simulink model "StateMachine_v3"  (R2015a)
settings: Solver=ode1  StartTime=0.0  StopTime=Inf  FixedStep=0.001  RelTol=1e-3
PostLoadFcn:
  | , if any(exist('dsrtsu_mdlpostloadfcn', 'file') == [2, 3, 6]), try dsrtsu_mdlpostloadfcn('Execute', bdroot); catch fprintf('Error in PostLoadFcn (dsrtsu_mdlpostloadfcn) for model "%s":\n %s\n', bdroot, lasterr); end, end,
libraries: rtican x25, rti1401lib_adc_type4 x16, rti1401lib_dio_type3 x16, rtilib1401 x1
(part 6 of 6)

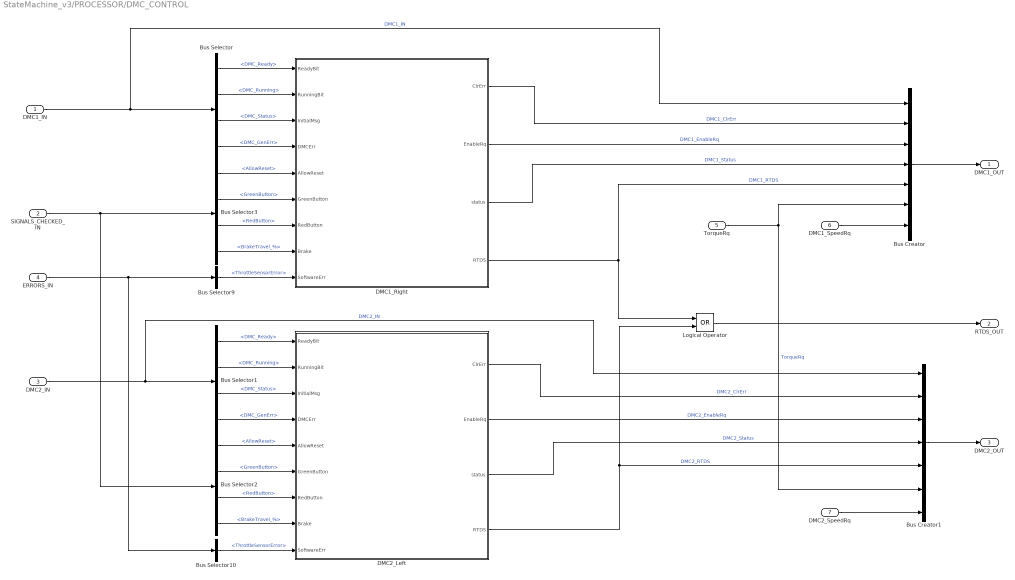
== system StateMachine_v3/PROCESSOR/DMC_CONTROL ==
  DMC1_IN : Inport
  SIGNALS_CHECKED_IN : Inport  Port=2
  DMC2_IN : Inport  Port=3
  ERRORS_IN : Inport  Port=4
  TorqueRq : Inport  Port=5
  DMC1_SpeedRq : Inport  Port=6
  DMC2_SpeedRq : Inport  Port=7
  Bus Creator : BusCreator  Inputs=7
  Bus Creator1 : BusCreator  Inputs=7
  Bus Selector : BusSelector  OutputSignals=DMC_Ready,DMC_Running,DMC_Status,DMC_GenErr
  Bus Selector1 : BusSelector  OutputSignals=DMC_Ready,DMC_Running,DMC_Status,DMC_GenErr
  Bus Selector10 : BusSelector  OutputSignals=ThrottleSensorError
  Bus Selector2 : BusSelector  OutputSignals=SIGNALS.OtherInputs.AllowReset,SIGNALS.DigitalInputs.GreenButton,SIGNALS.DigitalInputs.RedButton,BrakeTravel_%
  Bus Selector3 : BusSelector  OutputSignals=SIGNALS.OtherInputs.AllowReset,SIGNALS.DigitalInputs.GreenButton,SIGNALS.DigitalInputs.RedButton,BrakeTravel_%
  Bus Selector9 : BusSelector  OutputSignals=ThrottleSensorError
  DMC1_Right : Stateflow chart  TreatAsAtomicUnit=on
  DMC2_Left : Stateflow chart  TreatAsAtomicUnit=on
  Logical Operator : Logic  Operator=OR  AllPortsSameDT=off  OutDataTypeStr=boolean
  DMC1_OUT : Outport
  RTDS_OUT : Outport  Port=2
  DMC2_OUT : Outport  Port=3
  wires:
  TorqueRq/1 -> Bus Creator1/6, Bus Creator/6  "TorqueRq"
  ERRORS_IN/1 -> Bus Selector10/1, Bus Selector9/1
  SIGNALS_CHECKED_IN/1 -> Bus Selector2/1, Bus Selector3/1
  DMC1_Right/3(status) -> Bus Creator/4  "DMC1_Status"
  Bus Creator/1 -> DMC1_OUT/1
  Bus Selector9/1 -> DMC1_Right/9(SoftwareErr)  "<ThrottleSensorError>"
  Bus Selector10/1 -> DMC2_Left/9(SoftwareErr)  "<ThrottleSensorError>"
  Bus Creator1/1 -> DMC2_OUT/1
  Bus Selector/4 -> DMC1_Right/4(DMCErr)  "<DMC_GenErr>"
  Bus Selector3/3 -> DMC1_Right/7(RedButton)  "<RedButton>"
  DMC2_IN/1 -> Bus Creator1/1, Bus Selector1/1  "DMC2_IN"
  Bus Selector1/4 -> DMC2_Left/4(DMCErr)  "<DMC_GenErr>"
  DMC1_SpeedRq/1 -> Bus Creator/7
  DMC2_Left/3(status) -> Bus Creator1/4  "DMC2_Status"
  Bus Selector2/4 -> DMC2_Left/8(Brake)  "<BrakeTravel_%>"
  DMC2_Left/4(RTDS) -> Bus Creator1/5, Logical Operator/2  "DMC2_RTDS"
  DMC1_Right/4(RTDS) -> Logical Operator/1, Bus Creator/5  "DMC1_RTDS"
  Logical Operator/1 -> RTDS_OUT/1
  DMC2_Left/1(ClrErr) -> Bus Creator1/2  "DMC2_ClrErr"
  Bus Selector2/1 -> DMC2_Left/5(AllowReset)  "<AllowReset>"
  Bus Selector1/2 -> DMC2_Left/2(RunningBit)  "<DMC_Running>"
  DMC1_IN/1 -> Bus Creator/1, Bus Selector/1  "DMC1_IN"
  DMC1_Right/1(ClrErr) -> Bus Creator/2  "DMC1_ClrErr"
  DMC2_SpeedRq/1 -> Bus Creator1/7
  Bus Selector1/1 -> DMC2_Left/1(ReadyBit)  "<DMC_Ready>"
  Bus Selector3/2 -> DMC1_Right/6(GreenButton)  "<GreenButton>"
  Bus Selector/3 -> DMC1_Right/3(InitialMsg)  "<DMC_Status>"
  Bus Selector1/3 -> DMC2_Left/3(InitialMsg)  "<DMC_Status>"
  Bus Selector/1 -> DMC1_Right/1(ReadyBit)  "<DMC_Ready>"
  Bus Selector3/4 -> DMC1_Right/8(Brake)  "<BrakeTravel_%>"
  Bus Selector2/3 -> DMC2_Left/7(RedButton)  "<RedButton>"
  DMC2_Left/2(EnableRq) -> Bus Creator1/3  "DMC2_EnableRq"
  Bus Selector/2 -> DMC1_Right/2(RunningBit)  "<DMC_Running>"
  Bus Selector2/2 -> DMC2_Left/6(GreenButton)  "<GreenButton>"
  Bus Selector3/1 -> DMC1_Right/5(AllowReset)  "<AllowReset>"
  DMC1_Right/2(EnableRq) -> Bus Creator/3  "DMC1_EnableRq"

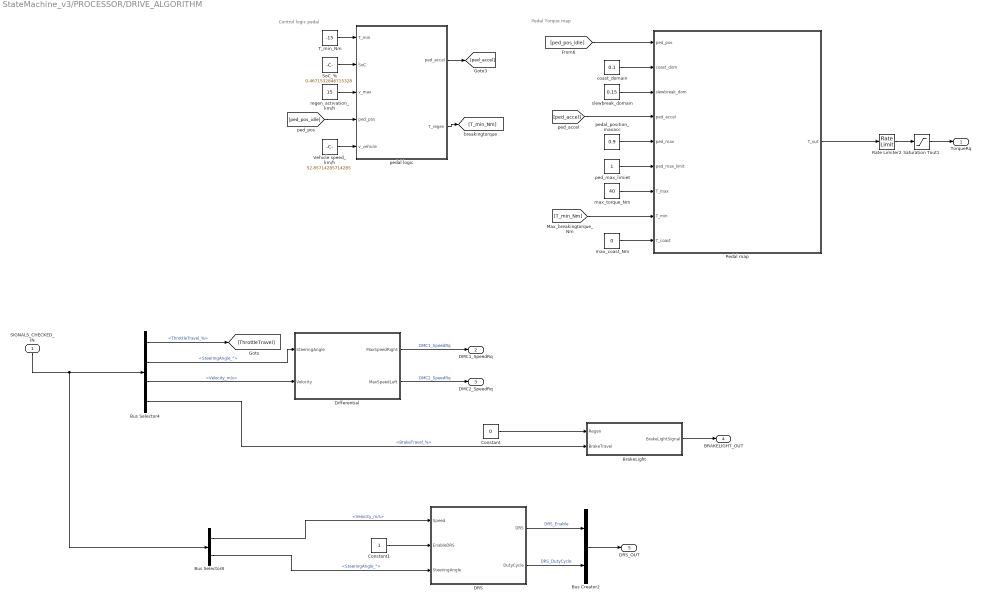
== system StateMachine_v3/PROCESSOR/DRIVE_ALGORITHM ==
  note: Control logic pedal
  note: Pedal Torque map
  SIGNALS_CHECKED_IN : Inport
  BrakeLight : MATLAB Function  TreatAsAtomicUnit=on
  Bus Creator2 : BusCreator  Inputs=2
  Bus Selector4 : BusSelector  OutputSignals=ThrottleTravel_%,SteeringAngle_°,Velocity_m/s,BrakeTravel_%
  Bus Selector8 : BusSelector  OutputSignals=Velocity_m/s,SteeringAngle_°
  Constant : Constant  Value=0
  Constant1 : Constant
  DRS : Stateflow chart  TreatAsAtomicUnit=on
  Differential : MATLAB Function  TreatAsAtomicUnit=on
  Pedal map : MATLAB Function  TreatAsAtomicUnit=on
  Rate Limiter2 : RateLimiter  RisingSlewLimit=20  FallingSlewLimit=-20  SampleTimeMode=inherited
  Saturation Tout1 : Saturate  UpperLimit=40  LowerLimit=-40
  SoC_% : Constant  Value=0.4671532846715328
  T_min_Nm : Constant  Value=-15
  Vehicle speed_km/h : Constant  Value=52.85714285714285
  coast_domain : Constant  Value=0.1
  max_coast_Nm : Constant  Value=0
  max_torque_Nm : Constant  Value=40
  ped_max_limiet : Constant
  pedal logic : Stateflow chart  TreatAsAtomicUnit=on
  pedal_position_maxacc : Constant  Value=0.9
  regen_activation_km/h : Constant  Value=15
  slewbreak_domain : Constant  Value=0.15
  TorqueRq : Outport
  DMC1_SpeedRq : Outport  Port=2
  DMC2_SpeedRq : Outport  Port=3
  BRAKELIGHT_OUT : Outport  Port=4
  DRS_OUT : Outport  Port=5
  wires:
  Bus Selector4/1 -> [ThrottleTravel]  "<ThrottleTravel_%>"
  Differential/2(MaxSpeedLeft) -> DMC2_SpeedRq/1  "DMC2_SpeedRq"
  Differential/1(MaxSpeedRight) -> DMC1_SpeedRq/1  "DMC1_SpeedRq"
  DRS/1(DRS) -> Bus Creator2/1  "DRS_Enable"
  BrakeLight/1(BrakeLightSignal) -> BRAKELIGHT_OUT/1
  DRS/2(DutyCycle) -> Bus Creator2/2  "DRS_DutyCycle"
  Bus Creator2/1 -> DRS_OUT/1
  Bus Selector4/2 -> Differential/1(SteeringAngle)  "<SteeringAngle_°>"
  Bus Selector4/3 -> Differential/2(Velocity)  "<Velocity_m/s>"
  Bus Selector8/2 -> DRS/3(SteeringAngle)  "<SteeringAngle_°>"
  Bus Selector8/1 -> DRS/1(Speed)  "<Velocity_m/s>"
  Bus Selector4/4 -> BrakeLight/2(BrakeTravel)  "<BrakeTravel_%>"
  Constant/1 -> BrakeLight/1(Regen)
  SIGNALS_CHECKED_IN/1 -> Bus Selector8/1, Bus Selector4/1
  Constant1/1 -> DRS/2(EnableDRS)
  Saturation Tout1/1 -> TorqueRq/1
  Pedal map/1(T_out) -> Rate Limiter2/1
  [ped_accel] -> Pedal map/4(ped_accel)
  Rate Limiter2/1 -> Saturation Tout1/1
  coast_domain/1 -> Pedal map/2(coast_dom)
  Vehicle speed_km/h/1 -> pedal logic/5(v_vehicle)
  [ped_pos_idle] -> pedal logic/4(ped_pos)
  pedal_position_maxacc/1 -> Pedal map/5(ped_max)
  T_min_Nm/1 -> pedal logic/1(T_min)
  ped_max_limiet/1 -> Pedal map/6(ped_max_limit)
  [ped_pos_idle] -> Pedal map/1(ped_pos)
  slewbreak_domain/1 -> Pedal map/3(slewbreak_dom)
  [T_min_Nm] -> Pedal map/8(T_min)
  SoC_%/1 -> pedal logic/2(SoC)
  pedal logic/2(T_regen) -> [T_min_Nm]
  max_torque_Nm/1 -> Pedal map/7(T_max)
  pedal logic/1(ped_accel) -> [ped_accel]
  regen_activation_km/h/1 -> pedal logic/3(v_max)
  max_coast_Nm/1 -> Pedal map/9(T_coast)

== system StateMachine_v3/RTI Data/RTI Data Store ==
  RTI Data Store : Subsystem  mask(RTI_DATA_STORE){}
      mask help:
      | RTI Data Store Block. This block is used by RTI to store internal model dependent data. Deleting this block will result in data loss.
      |
      | NEVER DELETE, COPY, OR MODIFY THIS BLOCK!
      mask Help:
      | RTI Data Store Block. This block is used by RTI to store internal model dependent data. Deleting this block will result in data loss.
      | 
      | NEVER DELETE, COPY, OR MODIFY THIS BLOCK!
      mask Display: text(0.5, 0.5, ' ', 'HorizontalAlignment', 'center');

== system StateMachine_v3/OUTPUT/DIGTIAL_OUTPUTS/DRS ==
  ServoFrequency : Inport
  Enable : EnablePort
  Divide : Product  Inputs=*/
  Gain : Gain  Gain=0.000001
  PWM DRS : rti1401lib_dio_type3/DIO_TYPE3_PWM_BL1  DSProperties=struct('RTI',struct('Version',uint32(2),'BlockType',struct('isSLSource',uint8(0),'isSLSink',uint8(1),'isHWSource',uint8(0),'isHWSink',uint8(1),'isSetup',uint8(0),'isInline',uint8(1),'isNonInline',uint8(0),'isInterrupt',uint8(0),'isChannelwise',uint8(1)),'IOBoardType',{{'DS1401','STD','DIOT3'}},'UnitType','PWM','Identifier','PWM','DialogType','ML','BlockSet','NONE','SlaveProcessor','NONE'))  RTIBlockInterface=struct('InputPortsWidth',int32([1 1]),'InputPortsActive',[1 1],'InputPortsName',{{'Period',['Duty Cycle']}},'BlockDisplay',{{['DIO TP3 PWM\nModule: 1\nPort: 1\nChannel: 7'],'center'}},'IconTransparency','on','InitLevel',3,'DialogFcn','rti1401stddiot3pwmgui','BlockName',struct('Token',{{'DIO_TYPE3_PWM_BL1'}}))  RTIBlockParameters=struct('ModuleNo',{{1,'OFF',[1 16]}},'PortNo',{{1,'OFF',[1 3]}},'ChannelNo',{{7,'OFF',[1 16]}},'SupplyRailsCh',{{[1 1],'OFF',[0 1 0 1]}},'UpdateMode',{{1,'ON',[1 2]}},'PeriodRange',{{7,'OFF',[1 16]}},'DutyCycleInit',{{'0','OFF',[0 1]}},'PeriodInit',{{'5e-05','OFF',[]}},'TerminationMode',{{0,'OFF',[0 1]}},'OutputTermValidate',{{0,'OFF',[0 1]}},'OutputTermBuildCheck',{{0,'OFF',[]}},'DutyCycleTerm',{{'0','OFF',[0 1]}},'PeriodTerm',{{'5e-05','OFF',[]}},'TLCFileName',{{'rti1401dio_t3_pwm','OFF',[]}},'EnableInterrupt',{{0,'OFF',[0 1]}},'TriggerEdgeType',{{1,'OFF',[1 3]}})  RTISFcnParameters=struct('ModuleNo','int32','PortNo','int16','ChannelNo','int16','SupplyRailsCh','int16','UpdateMode','int16','PeriodRange','int16','DutyCycleInit','double','PeriodInit','double','TerminationMode','int16','OutputTermValidate','int16','DutyCycleTerm','double','PeriodTerm','double','TLCFileName','char','EnableInterrupt','int16','TriggerEdgeType','int32')  RTIBlockParaDefault=struct('ModuleNo',1,'PortNo',1,'ChannelNo',1,'SupplyRailsCh',[1 1],'UpdateMode',1,'PeriodRange',7,'DutyCycleInit',0,'PeriodInit',5e-05,'TerminationMode',0,'OutputTermValidate',0,'OutputTermBuildCheck',0,'DutyCycleTerm',0,'PeriodTerm',5e-05,'TLCFileName','rti1401dio_t3_pwm','EnableInterrupt',0,'TriggerEdgeType',1)
  PWM DRS1 : rti1401lib_dio_type3/DIO_TYPE3_PWM_BL1  DSProperties=struct('RTI',struct('Version',uint32(2),'BlockType',struct('isSLSource',uint8(0),'isSLSink',uint8(1),'isHWSource',uint8(0),'isHWSink',uint8(1),'isSetup',uint8(0),'isInline',uint8(1),'isNonInline',uint8(0),'isInterrupt',uint8(0),'isChannelwise',uint8(1)),'IOBoardType',{{'DS1401','STD','DIOT3'}},'UnitType','PWM','Identifier','PWM','DialogType','ML','BlockSet','NONE','SlaveProcessor','NONE'))  RTIBlockInterface=struct('InputPortsWidth',int32([1 1]),'InputPortsActive',[1 1],'InputPortsName',{{'Period',['Duty Cycle']}},'BlockDisplay',{{['DIO TP3 PWM\nModule: 1\nPort: 1\nChannel: 8'],'center'}},'IconTransparency','on','InitLevel',3,'DialogFcn','rti1401stddiot3pwmgui','BlockName',struct('Token',{{'DIO_TYPE3_PWM_BL1'}}))  RTIBlockParameters=struct('ModuleNo',{{1,'OFF',[1 16]}},'PortNo',{{1,'OFF',[1 3]}},'ChannelNo',{{8,'OFF',[1 16]}},'SupplyRailsCh',{{[1 1],'OFF',[0 1 0 1]}},'UpdateMode',{{1,'ON',[1 2]}},'PeriodRange',{{7,'OFF',[1 16]}},'DutyCycleInit',{{'0','OFF',[0 1]}},'PeriodInit',{{'5e-05','OFF',[]}},'TerminationMode',{{0,'OFF',[0 1]}},'OutputTermValidate',{{0,'OFF',[0 1]}},'OutputTermBuildCheck',{{0,'OFF',[]}},'DutyCycleTerm',{{'0','OFF',[0 1]}},'PeriodTerm',{{'5e-05','OFF',[]}},'TLCFileName',{{'rti1401dio_t3_pwm','OFF',[]}},'EnableInterrupt',{{0,'OFF',[0 1]}},'TriggerEdgeType',{{1,'OFF',[1 3]}})  RTISFcnParameters=struct('ModuleNo','int32','PortNo','int16','ChannelNo','int16','SupplyRailsCh','int16','UpdateMode','int16','PeriodRange','int16','DutyCycleInit','double','PeriodInit','double','TerminationMode','int16','OutputTermValidate','int16','DutyCycleTerm','double','PeriodTerm','double','TLCFileName','char','EnableInterrupt','int16','TriggerEdgeType','int32')  RTIBlockParaDefault=struct('ModuleNo',1,'PortNo',1,'ChannelNo',1,'SupplyRailsCh',[1 1],'UpdateMode',1,'PeriodRange',7,'DutyCycleInit',0,'PeriodInit',5e-05,'TerminationMode',0,'OutputTermValidate',0,'OutputTermBuildCheck',0,'DutyCycleTerm',0,'PeriodTerm',5e-05,'TLCFileName','rti1401dio_t3_pwm','EnableInterrupt',0,'TriggerEdgeType',1)
  PeriodDRS : Constant  Value=0.008
  wires:
  PeriodDRS/1 -> Divide/2, PWM DRS1/1, PWM DRS/1
  ServoFrequency/1 -> Gain/1
  Divide/1 -> PWM DRS1/2, PWM DRS/2
  Gain/1 -> Divide/1

== system StateMachine_v3/RTI Data/RTI Data Store/RTI Data Store ==
  RTI Data Store : Subsystem  mask(RTI_DATA_STORE){}
      mask help:
      | RTI Data Store Block. This block is used by RTI to store internal model dependent data. Deleting this block will result in data loss.
      |
      | NEVER DELETE, COPY, OR MODIFY THIS BLOCK!
      mask Help:
      | RTI Data Store Block. This block is used by RTI to store internal model dependent data. Deleting this block will result in data loss.
      | 
      | NEVER DELETE, COPY, OR MODIFY THIS BLOCK!
      mask Display: text(0.5, 0.5, ' ', 'HorizontalAlignment', 'center');

== system StateMachine_v3/RTI Data/RTI Data Store/RTI Data Store/RTI Data Store ==
  RTI Data Store : Subsystem  mask(RTI_DATA_STORE){}
      mask help:
      | RTI Data Store Block. This block is used by RTI to store internal model dependent data. Deleting this block will result in data loss.
      |
      | NEVER DELETE, COPY, OR MODIFY THIS BLOCK!
      mask Help:
      | RTI Data Store Block. This block is used by RTI to store internal model dependent data. Deleting this block will result in data loss.
      | 
      | NEVER DELETE, COPY, OR MODIFY THIS BLOCK!
      mask Display: text(0.5, 0.5, ' ', 'HorizontalAlignment', 'center');

== system StateMachine_v3/RTI Data/RTI Data Store/RTI Data Store/RTI Data Store/RTI Data Store ==

== stateflow chart StateMachine_v3/PROCESSOR/DMC_CONTROL/DMC1_Right ==
  note: dSpace en DMC krijgen stroom doordat LV switch wordt omgedraaid
  state CheckCAN
    entry: status = 0;
    entry: EnableRq = 0;
    entry: ClrErr = 0;
    entry: RTDS = 0;
  note: Juiste bericht wordt opgesteld en voor de eerste keer verzonden door de dSpace
      | DMC zendt voor de eerste keer zijn berichten
  note: dSpace kijkt of hoe alle CAN berichten voor de eerste keer heeft ontvangen
  state InitialErrorClearing
    entry: status = 1;
    entry: EnableRq = 0;
    entry: ClrErr = 1;
  note: Alle berichten eens ontvangen, dus error clearen door van 0 -> 1 te zetten
  state Error
    entry: status = 2;
    entry: EnableRq = 0;
    entry: ClrErr = 0;
    entry: RTDS = 0;
  note: Conditie dat beide AIRs zijn gesloten
  note: Conditie dat beide AIRs zijn gesloten
  state ErrorFreeFrame
    state Offline
      entry: status = 4;
      entry: EnableRq = 0;
    state TimerOn
    state TimerOff
    state InitialisationRTD
      entry: status = 5;
      entry: EnableRq = 1;
      entry: ClrErr = 0;
      entry: RTDS = 1;
    state RTD
      entry: status = 6;
      entry: EnableRq = 1;
      entry: RTDS = 0;
    TimerOff -> Offline [order 2] : after(1,sec)
    Offline -> TimerOn : [ReadyBit == 1 && GreenButton == 1 && Brake > 50]
    TimerOn -> Offline [order 2] : [GreenButton == 0 || Brake < 50]
    TimerOn -> InitialisationRTD [order 1] : after (2,sec)
    TimerOff -> RTD [order 1] : [RedButton == 0]
    RTD -> TimerOff : [RedButton == 1]
    InitialisationRTD -> RTD : [RunningBit == 1 && after(2,sec)]
  state Reset
    entry: status = 3;
    entry: EnableRq = 0;
    entry: ClrErr = 1;
  (default) -> CheckCAN
  CheckCAN -> InitialErrorClearing : [InitialMsg == 1]
  InitialErrorClearing -> Error : [after(1,sec)]
  ErrorFreeFrame -> Error : [DMCErr == 1 || SoftwareErr == 1]
  Error -> Reset [order 2] : [AllowReset == 1 && (DMCErr == 1 || SoftwareErr == 1)]
  Error -> Offline [order 1] : [DMCErr == 0 && SoftwareErr ==0]
  Reset -> Offline
  data: ClrErr output; ReadyBit input; RunningBit input; InitialMsg input; DMCErr input; AllowReset input; GreenButton input; RedButton input; Brake input; EnableRq output; status output; RTDS output; SoftwareErr input

== matlab function StateMachine_v3/PRE-PROCESSOR/TemperatureConverter ==
  data: Vin input; u1 input; u2 input; u3 input; u4 input; u5 input; u6 input; y1 output; y2 output; y3 output; y4 output; y5 output; y6 output
function [y1,y2,y3,y4,y5,y6] = TemperatureConverter(Vin,u1,u2,u3,u4,u5,u6)

y1 = 3435/(log((u1*0.1)/(Vin-u1))+11.521046)-273.15;
y2 = 3435/(log((u2*0.1)/(Vin-u2))+11.521046)-273.15;
y3 = 3435/(log((u3*0.1)/(Vin-u3))+11.521046)-273.15;
y4 = 3435/(log((u4*0.1)/(Vin-u4))+11.521046)-273.15;
y5 = 3435/(log((u5*0.1)/(Vin-u5))+11.521046)-273.15;
y6 = 3435/(log((u5*0.1)/(Vin-u6))+11.521046)-273.15;

== stateflow chart StateMachine_v3/PROCESSOR/DMC_CONTROL/DMC2_Left ==
  note: dSpace en DMC krijgen stroom doordat LV switch wordt omgedraaid
  state CheckCAN
    entry: status = 0;
    entry: EnableRq = 0;
    entry: ClrErr = 0;
    entry: RTDS = 0;
  note: Juiste bericht wordt opgesteld en voor de eerste keer verzonden door de dSpace
      | DMC zendt voor de eerste keer zijn berichten
  note: dSpace kijkt of hoe alle CAN berichten voor de eerste keer heeft ontvangen
  state InitialErrorClearing
    entry: status = 1;
    entry: EnableRq = 0;
    entry: ClrErr = 1;
  note: Alle berichten eens ontvangen, dus error clearen door van 0 -> 1 te zetten
  state Error
    entry: status = 2;
    entry: EnableRq = 0;
    entry: ClrErr = 0;
    entry: RTDS = 0;
  note: Conditie dat beide AIRs zijn gesloten
  note: Conditie dat beide AIRs zijn gesloten
  state Reset
    entry: status = 3;
    entry: EnableRq = 0;
    entry: ClrErr = 1;
  state ErrorFreeFrame
    state Offline
      entry: status = 4;
      entry: EnableRq = 0;
    state TimerOn
    state TimerOff
    state InitialisationRTD
      entry: status = 5;
      entry: EnableRq = 1;
      entry: ClrErr = 0;
      entry: RTDS = 1;
    state RTD
      entry: status = 6;
      entry: EnableRq = 1;
      entry: RTDS = 0;
    TimerOff -> Offline [order 2] : after(1,sec)
    Offline -> TimerOn : [ReadyBit == 1 && GreenButton == 1 && Brake > 50]
    TimerOn -> Offline [order 2] : [GreenButton == 0 || Brake < 50]
    TimerOn -> InitialisationRTD [order 1] : after (2,sec)
    RTD -> TimerOff : [RedButton == 1]
    TimerOff -> RTD [order 1] : [RedButton == 0]
    InitialisationRTD -> RTD : [RunningBit == 1 && after(2,sec)]
  (default) -> CheckCAN
  CheckCAN -> InitialErrorClearing : [InitialMsg == 1]
  InitialErrorClearing -> Error : [after(1,sec)]
  ErrorFreeFrame -> Error : [DMCErr == 1 || SoftwareErr == 1]
  Error -> Reset [order 2] : [AllowReset == 1 && (DMCErr == 1 || SoftwareErr == 1)]
  Error -> Offline [order 1] : [DMCErr == 0 && SoftwareErr == 0]
  Reset -> Offline
  data: ClrErr output; ReadyBit input; RunningBit input; InitialMsg input; DMCErr input; AllowReset input; GreenButton input; RedButton input; Brake input; EnableRq output; status output; RTDS output; SoftwareErr input

== matlab function StateMachine_v3/PROCESSOR/DRIVE_ALGORITHM/BrakeLight ==
  data: Regen input; BrakeTravel input; BrakeLightSignal output
function BrakeLightSignal = BrakeLight(Regen,BrakeTravel)

if BrakeTravel > 0 || Regen == 1
    BrakeLightSignal = true;
else
    BrakeLightSignal = false;
end

== matlab function StateMachine_v3/PROCESSOR/DRIVE_ALGORITHM/Differential ==
  data: MaxSpeedRight output; MaxSpeedLeft output; SteeringAngle input; Velocity input
function [MaxSpeedRight,MaxSpeedLeft] = Differential(SteeringAngle, Velocity)
% Positive Turn = Right Turn

TrackWidth = 1.200; % d in m
TrackLength = 1.534; % L in m

TurnRadius =  TrackLength/tan(SteeringAngle*pi/180); % R in m
TurnSpeed = Velocity/TurnRadius; % Omega in rad/s
MaxSpeedRight = (TurnRadius - TrackWidth/2)*TurnSpeed; % V_r in m/s
MaxSpeedLeft = (TurnRadius + TrackWidth/2)*TurnSpeed; % V_l in m/s

== matlab function StateMachine_v3/PRE-PROCESSOR/MATLAB Function ==
  data: SteeringAngleTravel input; SteeringAngle output
function SteeringAngle = SteeringConverter(SteeringAngleTravel)

SteeringAngle = SteeringAngleTravel;

== matlab function StateMachine_v3/PRE-PROCESSOR/WSConverter ==
  data: WS_FR input; WS_FR_rpm output; WS_FL input; WS_RR input; WS_RL input; WS_FL_rpm output; WS_RR_rpm output; WS_RL_rpm output; Velocity_mps output; LongitudinalSlip output
function [WS_FR_rpm, WS_FL_rpm, WS_RR_rpm, WS_RL_rpm, Velocity_mps, LongitudinalSlip] = WSConverter(WS_FR, WS_FL, WS_RR, WS_RL)

NumberOfPulses = 46;
TireRadius = 0.4572/2;

WS_FR_rpm = WS_FR/NumberOfPulses*60;
WS_FL_rpm = WS_FL/NumberOfPulses*60;
WS_RR_rpm = WS_RR/NumberOfPulses*60;
WS_RL_rpm = WS_RL/NumberOfPulses*60;

WS_FR_mps = WS_FR_rpm*2*pi/60*TireRadius;
WS_FL_mps = WS_FL_rpm*2*pi/60*TireRadius;
WS_RR_mps = WS_RR_rpm*2*pi/60*TireRadius;
WS_RL_mps = WS_RL_rpm*2*pi/60*TireRadius;

Velocity_mps = (WS_FR_mps + WS_FL_mps)/2;
LongitudinalSlip = ((WS_RR_mps + WS_RL_mps)/2- Velocity_mps)/Velocity_mps;

== matlab function StateMachine_v3/PROCESSOR/DRIVE_ALGORITHM/Pedal map ==
  data: ped_pos input; coast_dom input; T_out output; slewbreak_dom input; ped_accel input; ped_max input; ped_max_limit input; T_max input; T_min input; T_coast input
function T_out = Pedalmap_eq(ped_pos,coast_dom,slewbreak_dom,ped_accel,ped_max,ped_max_limit,T_max,T_min,T_coast)
%%Accelerator pedal mapping:

ped_regen=ped_accel-coast_dom; %pedal postion - start regen - variable in function of velocity
ped_zero=ped_regen-slewbreak_dom; %pedal postion - start max regen - variable in function of velocity

slewrate_acc=(T_max-T_coast)/(ped_max-ped_accel); %slewrate acceleration region
slewrate_regen=(T_min-T_coast)/(ped_zero-ped_regen);%slewrate regen region

% acceleration pedal map eq.
T_out=T_min*(heavi(ped_pos,0)-heavi(ped_pos,ped_zero)) + (slewrate_regen*(ped_pos-ped_regen)+T_coast)*(heavi(ped_pos,ped_zero)-heavi(ped_pos,ped_regen))+T_coast*(heavi(ped_pos,ped_regen)-heavi(ped_pos,ped_accel))+(slewrate_acc*(ped_pos-ped_accel)+T_coast)*(heavi(ped_pos,ped_accel)-heavi(ped_pos,ped_max))+T_max*(heavi(ped_pos,ped_max-heavi(ped_pos,ped_max_limit)));

== matlab function StateMachine_v3/PRE-PROCESSOR/ThrottleSensorCalcuation ==
  data: e2 output; e1 output; u1 input; u2 input; y output
function [e2,e1,y] = ThrottleSensorCalculation(u1, u2)

% Variables
lowerlim1 = 0.33;
upperlim1 = 0.73;
lowerlim2 = 0.30;
upperlim2 = 0.70;

% ThrottleSensor1
t1 = 1-u1;
if t1 < lowerlim1
    y1 = 0;
elseif t1 > upperlim1
    y1 = 1;   
else
    y1 = (1/(upperlim1-lowerlim1))*(t1-lowerlim1);
end

% ThrottleSensor2
t2 = (1-u2);
if t2 < lowerlim2
    y2 = 0;
elseif t2 > upperlim2
    y2 = 1;   
else
    y2 = (1/(upperlim2-lowerlim2))*(t2-lowerlim2);
end

% ErrorCheck
if u1 > 0.10 && u1 < 0.90 && u2 > 0.10 && u2 < 0.90   
    if abs(y1-y2) > 0.10
        e1 = 1;
        e2 = 1;
        y = 0;
    else
        e1 = 0;
        e2 = 0;
        y = (y1+y2)/2;
    end
else
    if (u1 < 0.10 || u1 > 0.90) && (u2 < 0.10 || u2 > 0.90)
        e1 = 1;
        e2 = 1;
        y = 0;
    elseif u1 < 0.10 || u1 > 0.90
        e1 = 1;
        e2 = 0;
        y = y2;
    else
        e1 = 0;
        e2 = 1;
        y = y1;
    end  
    
%     e1 = 1;
%     e2 = 1;
%     y = 0;
end

== matlab function StateMachine_v3/PRE-PROCESSOR/BrakeSensorCalculation ==
  data: y output; u1 input; u2 input; e1 output; e2 output
function [y,e1,e2] = BrakeSensorCalculation(u1, u2)

% Variables
lowerlim1 = 0.33;
upperlim1 = 0.73;
lowerlim2 = 0.30;
upperlim2 = 0.70;

% BrakeeSensor1
t1 = (1-u1);
if t1 < lowerlim1
    y1 = 0;
elseif t1 > upperlim1
    y1 = 1;   
else
    y1 = (1/(upperlim1-lowerlim1))*(t1-lowerlim1);
end

% BrakeSensor2
t2 = (1-u2);
if t2 < lowerlim2
    y2 = 0;
elseif t2 > upperlim2
    y2 = 1;   
else
    y2 = (1/(upperlim2-lowerlim2))*(t2-lowerlim2);
end

% ErrorCheck
if u1 > 0.10 && u1 < 0.90 && u2 > 0.10 && u2 < 0.90   
    if abs(y1-y2) > 0.10
        e1 = 1;
        e2 = 1;
        y = 0;
    else
        e1 = 0;
        e2 = 0;
        y = (y1+y2)/2;
    end
else
    
    
    if (u1 < 0.10 || u1 > 0.90) && (u2 < 0.10 || u2 > 0.90)
        e1 = 1;
        e2 = 1;
        y = 0;
    elseif u1 < 0.10 || u1 > 0.90
        e1 = 1;
        e2 = 0;
        y = y2;
    else
        e1 = 0;
        e2 = 1;
        y = y1;
    end  
    
%     e1 = 1;
%     e2 = 1;
%     y = 0;
end

== stateflow chart StateMachine_v3/PROCESSOR/DRIVE_ALGORITHM/DRS ==
  state Offline
    entry: DRS = 0;
  state Standby
    entry:
    DRS = 1;
    DutyCycle = 900;
  state Online
    entry:
    DRS = 1;
    DutyCycle = 2100;
  (default) -> Offline
  Online -> Offline [order 2] : [EnableDRS == 0]
  Standby -> Offline [order 1] : [EnableDRS == 0]
  Offline -> Standby : [EnableDRS == 1]
  Online -> Standby [order 1] : [Speed < 10 || abs(SteeringAngle) < 10 ]
  Standby -> Online [order 2] : [Speed > 15 && abs(SteeringAngle) > 15]
  data: Speed input; EnableDRS input; DRS output; DutyCycle output; SteeringAngle input

== stateflow chart StateMachine_v3/PROCESSOR/DRIVE_ALGORITHM/pedal logic ==
  state Driving
    state Disable_regen %SoC is to high.
      entry:
      ped_accel=0.45;
      T_regen=0;
    state Activate_regen
      entry:
      ped_accel=0.45;
      T0= -5; %Regentorque at v_max [Nm]
      during:
      % velocity dependant braking torque
      if v_vehicle<15
      T_regen=T_min/15
      elseif v_vehicle<50
      T_regen=T_min
      else
      T_regen=(T_min-T0)/(50-100)*(v_vehicle-100)+T0
      end
    (default) -> Disable_regen %SoC is to high.
    Disable_regen %SoC is to high. -> Activate_regen : [SoC<0.95]
    Activate_regen -> Disable_regen %SoC is to high. : [SoC>0.95]
  state Standstill
    entry:
    T_regen=0;
    ped_accel=0.1; %
    during:
    %velocity dependent coasting until v_max
    if ped_pos>0.1
    ped_accel=min(ped_pos* (v_vehicle/v_max),0.45); %Offset of 0.1
    end
    exit:
    ped_accel=0.45;
  (default) -> Standstill
  Driving -> Standstill : [v_vehicle<=5]
  Standstill -> Driving : [v_vehicle >v_max&&ped_pos>0.45]
  data: T_min input; SoC input; v_max input; ped_pos input; v_vehicle input; ped_accel output; T_regen output; T0 local
